simulink model "Modell_PADDELEC_RB_V3"  (R2019b)
settings: Solver=FixedStepAuto  StartTime=0.0  StopTime=269.98659999999654  FixedStep=0.1  RelTol=1e-3
model workspace (MAT data in the model file):
  SDO_OutputTimes = [0 0.00219999999536 0.0177999999942 0.0334999999977 0.0399999999936 0.0490999999965 0.0497999999934 0.0646999999954 0.0799999999945 0.0802999999942 0.0959000000003 0.111599999997 ... (25110 elements, 25110x1)]
values from neighbouring files (symbols this model uses):
  BAT = clsBattery    [start.m]
  BLDC = clsBLDC    [start.m]
  BoatHull = clsBoatHull    [start.m]
  MotorECU = clsMotorECU    [start.m]
libraries: fl_lib x51, nesl_utility x28, ee_lib x3, simulink x2, eeGeneralControl x1
(part 2 of 2)

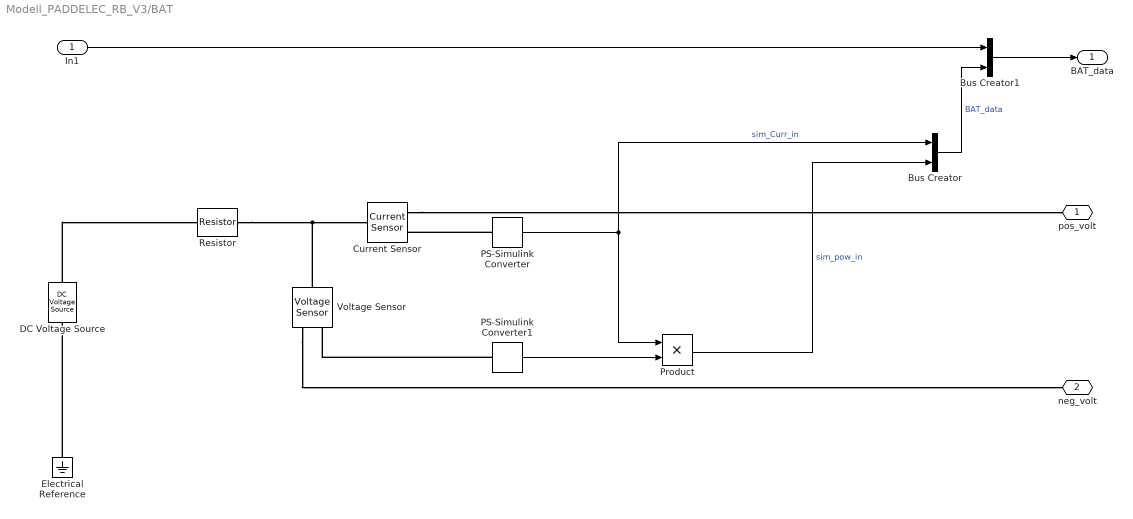
== system Modell_PADDELEC_RB_V3/BAT ==
  In1 : Inport
  Bus Creator : BusCreator  Inputs=2
  Bus Creator1 : BusCreator  Inputs=2
  Current Sensor : fl_lib/Electrical/Electrical Sensors/Current Sensor
  DC Voltage Source : fl_lib/Electrical/Electrical Sources/DC Voltage Source  v0=BAT.Voltage V
  Electrical Reference : fl_lib/Electrical/Electrical Elements/Electrical Reference
  PS-Simulink Converter : nesl_utility/PS-Simulink Converter  PhysicalDomain=network_engine_domain  SubClassName=ps_output  LeftPortType=input  RightPortType=output  PseudoPeriodic=off  Frequencies=[]  Unit=1  AffineConversion=off
  PS-Simulink Converter1 : nesl_utility/PS-Simulink Converter  PhysicalDomain=network_engine_domain  SubClassName=ps_output  LeftPortType=input  RightPortType=output  PseudoPeriodic=off  Frequencies=[]  Unit=1  AffineConversion=off
  Product : Product
  Resistor : fl_lib/Electrical/Electrical Elements/Resistor  R=BAT.InternalResistance Ohm  i_specify=off  i_priority=High  i=0 A  i_nominal_specify=off  i_nominal_unit=A  i_nominal_value=1  v_specify=off  v_priority=High  v=0 V  v_nominal_specify=off  v_nominal_unit=V  v_nominal_value=1
  Voltage Sensor : fl_lib/Electrical/Electrical Sensors/Voltage Sensor
  pos_volt : PMIOPort  Side=Right
  neg_volt : PMIOPort  Port=2  Side=Right
  BAT_data : Outport
  wires:
  PS-Simulink Converter/1 -> Product/1, Bus Creator/1  "sim_Curr_in"
  Product/1 -> Bus Creator/2  "sim_pow_in"
  PS-Simulink Converter1/1 -> Product/2
  Bus Creator1/1 -> BAT_data/1
  Bus Creator/1 -> Bus Creator1/2  "BAT_data"
  In1/1 -> Bus Creator1/1
  connections:
  Electrical Reference/LConn1 -- DC Voltage Source/RConn1
  Voltage Sensor/LConn1 -- Current Sensor/LConn1 -- Resistor/RConn1
  PS-Simulink Converter1/LConn1 -- Voltage Sensor/RConn1
  PS-Simulink Converter/LConn1 -- Current Sensor/RConn1
  DC Voltage Source/LConn1 -- Resistor/LConn1
  Voltage Sensor/RConn2 -- neg_volt/RConn1
  Current Sensor/RConn2 -- pos_volt/RConn1

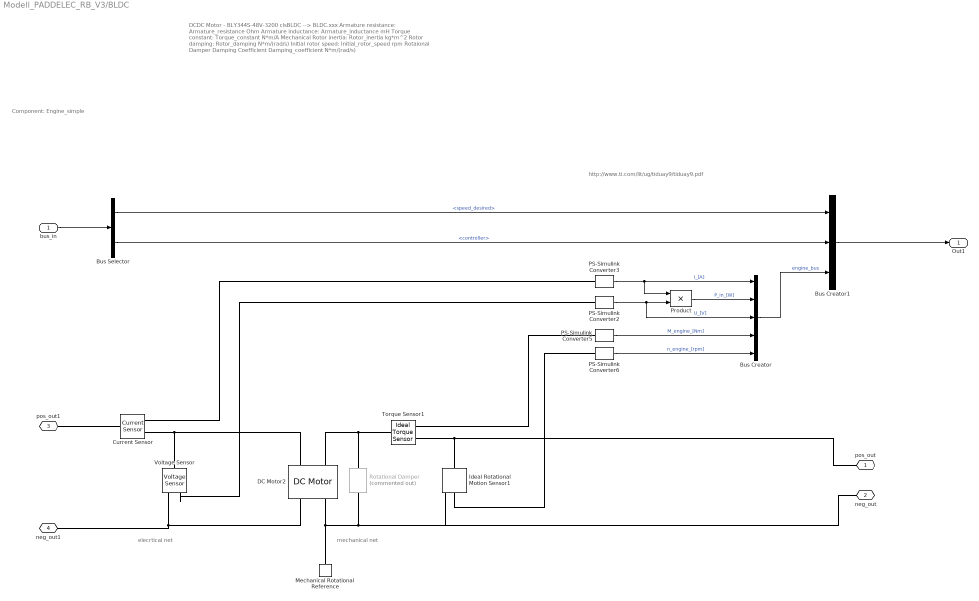
== system Modell_PADDELEC_RB_V3/BLDC ==
  note: http://www.ti.com/lit/ug/tiduay9/tiduay9.pdf
  note: mechanical net
  note: DCDC Motor - BLY344S-48V-3200
      |
      | clsBLDC --> BLDC.xxx
      |
      | Armature resistance:
      | Armature_resistance
      | Ohm
      |
      | Armature inductance:
      | Armature_inductance
      | mH
      |
      | Torque constant:
      | Torque_constant
      | N*m/A
      |
      | Mechanical
      |
      | Rotor inertia:
      | Rotor_inertia
      | kg*m^2
      |
      | Rotor damping:
      | Rotor_damping
      | N*m/(rad/s)
      |
      | Initial rotor speed:
      | Initial_rotor_speed
      | rpm
      |
      | Rotaional Damper
      |
      | Damping Coefficient
      | Damping_coefficient
      | N*m/(rad/s)
  note: elecrtical net
  note: Component:
      | Engine_simple
  bus_in : Inport
  Bus Creator : BusCreator  Inputs=5
  Bus Creator1 : BusCreator  Inputs=3
  Bus Selector : BusSelector  OutputSignals=speed_desired,controller
  Current Sensor : fl_lib/Electrical/Electrical Sensors/Current Sensor
  DC Motor2 : ee_lib/Electromechanical/Brushed Motors/DC Motor  parameterization=1  Ra=BLDC.Armature_resistance Ohm  La=BLDC.Armature_inductance mH  emf_or_torque=2  Kv=0.00907 V/rpm  Ki=BLDC.Torque_constant N*m/A  T_stall=3e-3*4000/(2*pi*6.25) N*m  w_max=3200 rpm  w_rated=3200 rpm  P_rated=660 W  V_rated=48 V  J="BLDC.Rotor_inertia  kg*m^2"  lam_param=1  lam=BLDC.Rotor_damping N*m/(rad/s)  i_noload=0 A  V_i_noload=1.5 V  speed0=BLDC.Initial_rotor_speed rpm  alpha=3.93e-3 1/K  Tmeas=25 degC  thermal_mass=100 J/K  initial_temperature=25 degC
      settings: SourceProductName=Simscape Electrical
  Ideal Rotational Motion Sensor1 : fl_lib/Mechanical/Mechanical Sensors/Ideal Rotational Motion Sensor  offset=0 rad
  Mechanical Rotational Reference : fl_lib/Mechanical/Rotational Elements/Mechanical Rotational Reference
  PS-Simulink Converter2 : nesl_utility/PS-Simulink Converter  PhysicalDomain=network_engine_domain  SubClassName=ps_output  LeftPortType=input  RightPortType=output  PseudoPeriodic=off  Frequencies=[]  Unit=V  AffineConversion=off
  PS-Simulink Converter3 : nesl_utility/PS-Simulink Converter  PhysicalDomain=network_engine_domain  SubClassName=ps_output  LeftPortType=input  RightPortType=output  PseudoPeriodic=off  Frequencies=[]  Unit=A  AffineConversion=off
  PS-Simulink Converter5 : nesl_utility/PS-Simulink Converter  PhysicalDomain=network_engine_domain  SubClassName=ps_output  LeftPortType=input  RightPortType=output  PseudoPeriodic=off  Frequencies=[]  Unit=N*m  AffineConversion=on
  PS-Simulink Converter6 : nesl_utility/PS-Simulink Converter  PhysicalDomain=network_engine_domain  SubClassName=ps_output  LeftPortType=input  RightPortType=output  PseudoPeriodic=off  Frequencies=[]  Unit=rpm  AffineConversion=on
  Product : Product
  Rotational Damper : fl_lib/Mechanical/Rotational Elements/Rotational Damper  Commented=on  D=2.5000e-04 N*m/(rad/s)  w_specify=off  w_priority=High  w=0 rad/s  w_nominal_specify=off  w_nominal_unit=rad/s  w_nominal_value=1  t_specify=off  t_priority=High  t=0 N*m  t_nominal_specify=off  t_nominal_unit=N*m  t_nominal_value=1
  Torque Sensor1 : fl_lib/Mechanical/Mechanical Sensors/Ideal Torque Sensor
  Voltage Sensor : fl_lib/Electrical/Electrical Sensors/Voltage Sensor
  pos_out : PMIOPort  Side=Right
  neg_out : PMIOPort  Port=2  Side=Right
  pos_out1 : PMIOPort  Port=3  Side=Left
  neg_out1 : PMIOPort  Port=4  Side=Left
  Out1 : Outport
  wires:
  Bus Creator1/1 -> Out1/1
  Bus Selector/2 -> Bus Creator1/2  "<controller>"
  Product/1 -> Bus Creator/2  "P_in_[W]"
  PS-Simulink Converter3/1 -> Bus Creator/1, Product/1  "I_[A]"
  bus_in/1 -> Bus Selector/1
  PS-Simulink Converter2/1 -> Bus Creator/3, Product/2  "U_[V]"
  Bus Creator/1 -> Bus Creator1/3  "engine_bus"
  PS-Simulink Converter5/1 -> Bus Creator/4  "M_engine_[Nm]"
  PS-Simulink Converter6/1 -> Bus Creator/5  "n_engine_[rpm]"
  Bus Selector/1 -> Bus Creator1/1  "<speed_desired>"
  connections:
  DC Motor2/RConn1 -- Voltage Sensor/RConn2 -- neg_out1/RConn1
  Torque Sensor1/RConn1 -- Ideal Rotational Motion Sensor1/LConn1 -- pos_out/RConn1
  DC Motor2/RConn2 -- Rotational Damper/RConn1 -- neg_out/RConn1 -- Ideal Rotational Motion Sensor1/RConn1 -- Mechanical Rotational Reference/LConn1
  DC Motor2/LConn2 -- Torque Sensor1/LConn1 -- Rotational Damper/LConn1
  DC Motor2/LConn1 -- Current Sensor/RConn2 -- Voltage Sensor/LConn1
  Ideal Rotational Motion Sensor1/RConn2 -- PS-Simulink Converter6/LConn1
  Torque Sensor1/RConn2 -- PS-Simulink Converter5/LConn1
  pos_out1/RConn1 -- Current Sensor/LConn1
  Voltage Sensor/RConn1 -- PS-Simulink Converter2/LConn1
  Current Sensor/RConn1 -- PS-Simulink Converter3/LConn1

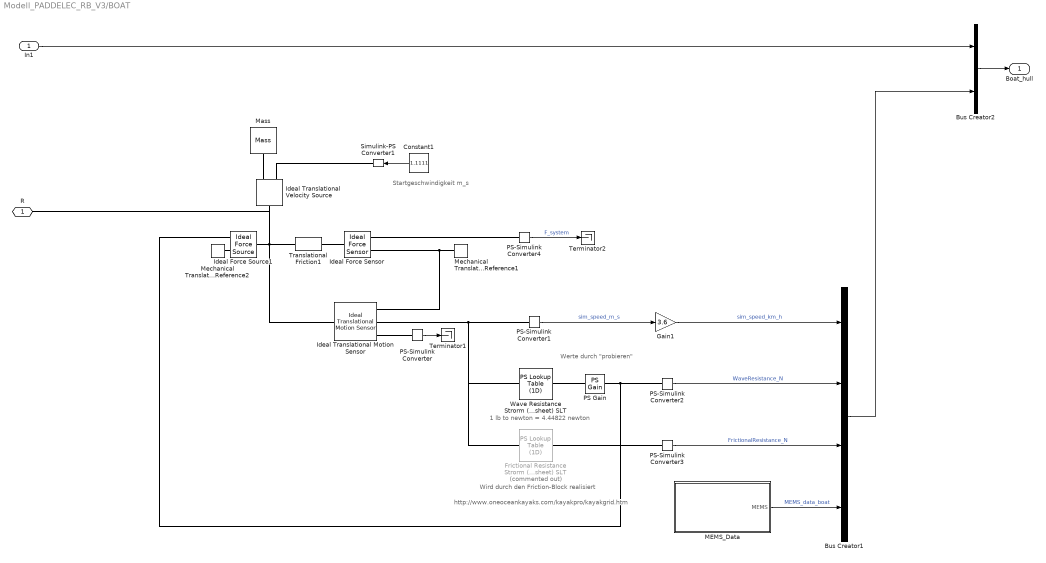
== system Modell_PADDELEC_RB_V3/BOAT ==
  note: Startgeschwindigkeit m_s
  note: Wird durch den Friction-Block realisiert
  note: 1 lb to newton = 4.44822 newton
  note: http://www.oneoceankayaks.com/kayakpro/kayakgrid.htm
  note: Werte durch "probieren"
  In1 : Inport
  Bus Creator1 : BusCreator  Inputs=4
  Bus Creator2 : BusCreator  Inputs=2
  Constant1 : Constant  Value=1.1111
  Frictional Resistance Strorm (datasheet) SLT : fl_lib/Physical Signals/Lookup Tables/PS Lookup Table (1D)  Commented=on  x=SpeedVec_m_s m/s  f=FricResistance_N  interp_method=simscape.enum.interpolation.smooth  extrap_method=simscape.enum.extrapolation.linear
      settings: SourceProductName=Simscape  SourceProductBaseCode=SS
  Gain1 : Gain  Gain=3.6
  Ideal Force Sensor : fl_lib/Mechanical/Mechanical Sensors/Ideal Force Sensor
  Ideal Force Source1 : fl_lib/Mechanical/Mechanical Sources/Ideal Force Source
  Ideal Translational Motion Sensor : fl_lib/Mechanical/Mechanical Sensors/Ideal Translational Motion Sensor  offset=0 m
  Ideal Translational Velocity Source : fl_lib/Mechanical/Mechanical Sources/Ideal Translational Velocity Source
  MEMS_Data : Subsystem
      mask Display: image('D:\00_Sandbox\Matlab\Modell_20200324\03_symbols\Lagesensoren.png'); % Use "Edit Image" on toolstrip to change.
  Mass : fl_lib/Mechanical/Translational Elements/Mass  mass=BoatHull.Mass + 195.5 kg  v_specify=off  v_priority=High  v=0 m/s  v_nominal_specify=off  v_nominal_unit=m/s  v_nominal_value=1  f_specify=off  f_priority=None  f=0 N  f_nominal_specify=off  f_nominal_unit=N  f_nominal_value=1
  Mechanical Translational Reference1 : fl_lib/Mechanical/Translational Elements/Mechanical Translational Reference
  Mechanical Translational Reference2 : fl_lib/Mechanical/Translational Elements/Mechanical Translational Reference
  PS Gain : fl_lib/Physical Signals/Functions/PS Gain  gain=-32
  PS-Simulink Converter : nesl_utility/PS-Simulink Converter  PhysicalDomain=network_engine_domain  SubClassName=ps_output  LeftPortType=input  RightPortType=output  PseudoPeriodic=off  Frequencies=[]  Unit=inherit  AffineConversion=off
  PS-Simulink Converter1 : nesl_utility/PS-Simulink Converter  PhysicalDomain=network_engine_domain  SubClassName=ps_output  LeftPortType=input  RightPortType=output  PseudoPeriodic=off  Frequencies=[]  Unit=inherit  AffineConversion=off
  PS-Simulink Converter2 : nesl_utility/PS-Simulink Converter  PhysicalDomain=network_engine_domain  SubClassName=ps_output  LeftPortType=input  RightPortType=output  PseudoPeriodic=off  Frequencies=[]  Unit=inherit  AffineConversion=on
  PS-Simulink Converter3 : nesl_utility/PS-Simulink Converter  PhysicalDomain=network_engine_domain  SubClassName=ps_output  LeftPortType=input  RightPortType=output  PseudoPeriodic=off  Frequencies=[]  Unit=inherit  AffineConversion=on
  PS-Simulink Converter4 : nesl_utility/PS-Simulink Converter  PhysicalDomain=network_engine_domain  SubClassName=ps_output  LeftPortType=input  RightPortType=output  PseudoPeriodic=off  Frequencies=[]  Unit=inherit  AffineConversion=off
  Simulink-PS Converter1 : nesl_utility/Simulink-PS Converter  PhysicalDomain=network_engine_domain  SubClassName=ps_input  LeftPortType=input  RightPortType=output  PseudoPeriodic=off  Frequencies=[]  NoiseDistribution=none  NoiseParameters=[]  Unit=1  AffineConversion=off  FilteringAndDerivatives=provide  SimscapeFilterOrder=1  InputFilterTimeConstant=0.001  UdotUserProvided=0
  Terminator1 : Terminator
  Terminator2 : Terminator
  Translational Friction1 : fl_lib/Mechanical/Translational Elements/Translational Friction  brkwy_frc=BoatHull.BreakawayFrictionForce N  brkwy_vel=BoatHull.BreakawayFrictionVelocity m/s  Col_frc=BoatHull.ColumbFrictionForce N  visc_coef=BoatHull.ViscousFriction N/(m/s)  v_specify=off  v_priority=None  v=0 m/s  v_nominal_specify=off  v_nominal_unit=m/s  v_nominal_value=1  f_specify=off  f_priority=None  f=0 N  f_nominal_specify=off  f_nominal_unit=N  f_nominal_value=1
      settings: SourceProductName=Simscape  SourceProductBaseCode=SS  InternalSimscapePortConfiguration="{\"Bottom\":[],\"Left\":[{\"id\":\"R\",\"label\":\"R\",\"type\":\"foundation.mechanical.translational.translational\"}],\"Right\":[{\"id\":\"C\",\"label\":\"C\",\"type\":\"foundation.mechanical.translational.translational\"}],\"Top\":[]}"
  Wave Resistance Strorm (datasheet) SLT : fl_lib/Physical Signals/Lookup Tables/PS Lookup Table (1D)  x=BoatHull.SpeedVec_m_s m/s  f=BoatHull.WaveResistance_N  interp_method=simscape.enum.interpolation.smooth  extrap_method=simscape.enum.extrapolation.linear
      settings: SourceProductName=Simscape  SourceProductBaseCode=SS
  R : PMIOPort  Side=Left
  Boat_hull : Outport  VectorParamsAs1DForOutWhenUnconnected=off
  wires:
  PS-Simulink Converter/1 -> Terminator1/1
  PS-Simulink Converter2/1 -> Bus Creator1/2  "WaveResistance_N"
  Gain1/1 -> Bus Creator1/1  "sim_speed_km_h"
  PS-Simulink Converter1/1 -> Gain1/1  "sim_speed_m_s"
  PS-Simulink Converter3/1 -> Bus Creator1/3  "FrictionalResistance_N"
  PS-Simulink Converter4/1 -> Terminator2/1  "F_system"
  Constant1/1 -> Simulink-PS Converter1/1
  MEMS_Data/1(MEMS) -> Bus Creator1/4  "MEMS_data_boat"
  In1/1 -> Bus Creator2/1
  Bus Creator1/1 -> Bus Creator2/2
  Bus Creator2/1 -> Boat_hull/1
  connections:
  Ideal Translational Motion Sensor/LConn1 -- R/RConn1 -- Ideal Translational Velocity Source/LConn1 -- Ideal Force Source1/LConn1 -- Translational Friction1/LConn1
  Ideal Translational Motion Sensor/RConn1 -- Mechanical Translational Reference1/LConn1 -- Ideal Force Sensor/RConn1
  PS-Simulink Converter/LConn1 -- Ideal Translational Motion Sensor/RConn3
  Ideal Translational Motion Sensor/RConn2 -- Frictional Resistance Strorm (datasheet) SLT/LConn1 -- Wave Resistance Strorm (datasheet) SLT/LConn1 -- PS-Simulink Converter1/LConn1
  PS-Simulink Converter3/LConn1 -- Frictional Resistance Strorm (datasheet) SLT/RConn1
  PS-Simulink Converter2/LConn1 -- Ideal Force Source1/RConn1 -- PS Gain/RConn1
  PS Gain/LConn1 -- Wave Resistance Strorm (datasheet) SLT/RConn1
  PS-Simulink Converter4/LConn1 -- Ideal Force Sensor/RConn2
  Ideal Force Sensor/LConn1 -- Translational Friction1/RConn1
  Simulink-PS Converter1/RConn1 -- Ideal Translational Velocity Source/RConn1
  Ideal Translational Velocity Source/RConn2 -- Mass/LConn1
  Mechanical Translational Reference2/LConn1 -- Ideal Force Source1/RConn2

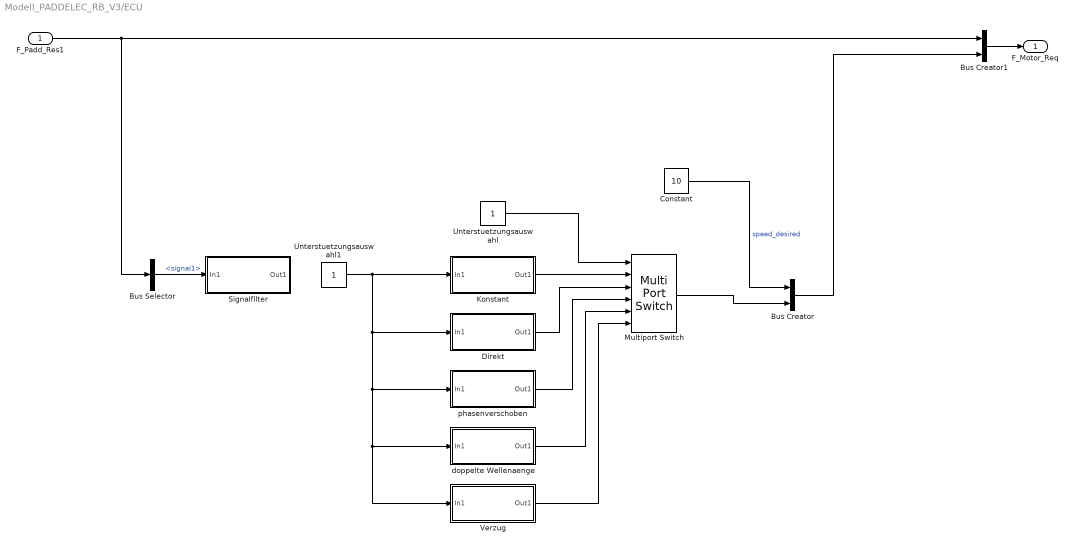
== system Modell_PADDELEC_RB_V3/ECU ==
  F_Padd_Res1 : Inport
  Bus Creator : BusCreator  Inputs=2
  Bus Creator1 : BusCreator  Inputs=2
  Bus Selector : BusSelector  OutputSignals=signal1
  Constant : Constant  Value=10
  Direkt : Subsystem
  Konstant : Subsystem
  Multiport Switch : MultiPortSwitch  Inputs=5
  Signalfilter : Subsystem
  Unterstuetzungsauswahl : Constant
  Unterstuetzungsauswahl1 : Constant
  Verzug : Subsystem
  doppelte Wellenaenge : Subsystem
  phasenverschoben : Subsystem
  F_Motor_Req : Outport  VectorParamsAs1DForOutWhenUnconnected=off
  wires:
  Konstant/1(Out1) -> Multiport Switch/2
  Unterstuetzungsauswahl1/1 -> Verzug/1(In1), doppelte Wellenaenge/1(In1), phasenverschoben/1(In1), Direkt/1(In1), Konstant/1(In1)
  Direkt/1(Out1) -> Multiport Switch/3
  Unterstuetzungsauswahl/1 -> Multiport Switch/1
  phasenverschoben/1(Out1) -> Multiport Switch/4
  doppelte Wellenaenge/1(Out1) -> Multiport Switch/5
  Verzug/1(Out1) -> Multiport Switch/6
  Constant/1 -> Bus Creator/1  "speed_desired"
  Multiport Switch/1 -> Bus Creator/2
  F_Padd_Res1/1 -> Bus Creator1/1, Bus Selector/1
  Bus Creator/1 -> Bus Creator1/2
  Bus Creator1/1 -> F_Motor_Req/1
  Bus Selector/1 -> Signalfilter/1(In1)  "<signal1>"

== system Modell_PADDELEC_RB_V3/JET  ==
  n_Motor : Inport
  Mechanical Rotational Reference : fl_lib/Mechanical/Rotational Elements/Mechanical Rotational Reference
  Slider-Crank : fl_lib/Mechanical/Mechanisms/Slider-Crank  crank=.1 m  rod=.2 m  inertia=0.01 kg*m^2  k=1e6 N/m  b=1e3 N/(m/s)  theta_specify=off  theta_priority=High  theta=1.570796326794897 rad  theta_nominal_specify=off  theta_nominal_unit=rad  theta_nominal_value=1  w_specify=off  w_priority=High  w=0 rad/s  w_nominal_specify=off  w_nominal_unit=rad/s  w_nominal_value=1
      settings: SourceProductName=Simscape  SourceProductBaseCode=SS  InternalSimscapePortConfiguration="{\"Bottom\":[],\"Left\":[{\"id\":\"C\",\"label\":\"C\",\"type\":\"foundation.mechanical.rotational.rotational\"}],\"Right\":[{\"id\":\"S\",\"label\":\"S\",\"type\":\"foundation.mechanical.translational.translational\"}],\"Top\":[]}"
  pos_in : PMIOPort  Side=Left
  R : PMIOPort  Port=2  Side=Right
  neg_in : PMIOPort  Port=3  Side=Left
  F_Jet : Outport
  wires:
  n_Motor/1 -> F_Jet/1
  connections:
  pos_in/RConn1 -- Slider-Crank/LConn1
  Slider-Crank/RConn1 -- R/RConn1
  neg_in/RConn1 -- Mechanical Rotational Reference/LConn1

== system Modell_PADDELEC_RB_V3/Messungen ==
  Bus Creator : BusCreator  Inputs=2
  From Workspace1 : FromWorkspace  VariableName=tsc_paddel4.scaledAccelX  SampleTime=0
  From Workspace2 : FromWorkspace  VariableName=tsc_paddel4.speed  SampleTime=0
  Gain : Gain  Gain=-1
  Gain1 : Gain  Gain=3.6
  measurement_data : Outport
  wires:
  From Workspace1/1 -> Gain/1
  Gain/1 -> Bus Creator/1  "a_Boat"
  From Workspace2/1 -> Gain1/1  "v_Boat"
  Bus Creator/1 -> measurement_data/1
  Gain1/1 -> Bus Creator/2  "v_Boat_km_h"

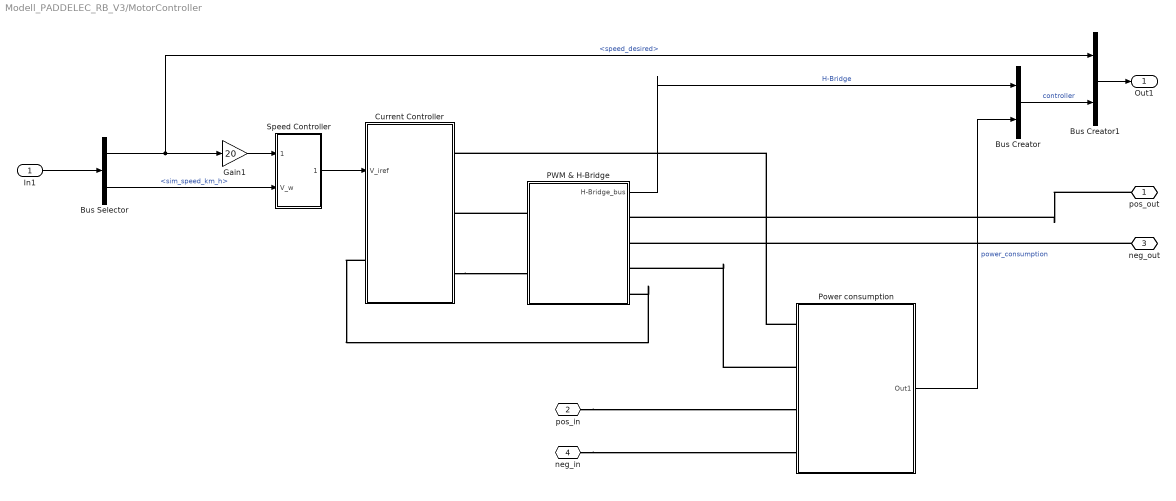
== system Modell_PADDELEC_RB_V3/MotorController ==
  In1 : Inport
  Bus Creator : BusCreator  Inputs=2
  Bus Creator1 : BusCreator  Inputs=2
  Bus Selector : BusSelector  OutputSignals=signal1.signal2.speed_desired,signal1.signal1.signal1.signal2.sim_speed_km_h
  Current Controller : Subsystem
  Gain1 : Gain  Gain=20
  PWM & H-Bridge : Subsystem
  Power consumption : Subsystem
  Speed Controller : Subsystem  VariantControl=VSS_SpeedController_simple
  pos_out : PMIOPort  Side=Right
  pos_in : PMIOPort  Port=2  Side=Left
  neg_out : PMIOPort  Port=3  Side=Right
  neg_in : PMIOPort  Port=4  Side=Left
  Out1 : Outport
  wires:
  In1/1 -> Bus Selector/1
  Power consumption/1(Out1) -> Bus Creator/2  "power_consumption"
  Gain1/1 -> Speed Controller/1(V_wref)
  Bus Creator1/1 -> Out1/1
  Bus Selector/2 -> Speed Controller/2(V_w)  "<sim_speed_km_h>"
  Speed Controller/1(V_iref) -> Current Controller/1(V_iref)
  PWM & H-Bridge/1(H-Bridge_bus) -> Bus Creator/1  "H-Bridge"
  Bus Creator/1 -> Bus Creator1/2  "controller"
  Bus Selector/1 -> Gain1/1, Bus Creator1/1  "<speed_desired>"
  connections:
  neg_out/RConn1 -- PWM & H-Bridge/RConn2
  PWM & H-Bridge/LConn1 -- Current Controller/RConn2
  Current Controller/RConn3 -- PWM & H-Bridge/LConn2
  pos_out/RConn1 -- PWM & H-Bridge/RConn1
  Power consumption/LConn2 -- PWM & H-Bridge/RConn3
  Power consumption/LConn1 -- Current Controller/RConn1
  Current Controller/LConn1 -- PWM & H-Bridge/RConn4
  pos_in/RConn1 -- Power consumption/LConn3
  neg_in/RConn1 -- Power consumption/LConn4

== system Modell_PADDELEC_RB_V3/Subsystem1 ==
  a_Boat_sim : Inport
  In4 : Inport  Port=2
  Bus Selector : BusSelector  OutputSignals=signal2.sim_speed_km_h,signal2.WaveResistance_N
  Bus Selector1 : BusSelector  OutputSignals=a_Boat,v_Boat_km_h
  v_Boat : Scope  NumInputPorts=2
  v_Boat1 : Scope  NumInputPorts=2
  wires:
  a_Boat_sim/1 -> Bus Selector/1
  In4/1 -> Bus Selector1/1
  Bus Selector/1 -> v_Boat/1  "<sim_speed_km_h>"
  Bus Selector/2 -> v_Boat/2  "<WaveResistance_N>"
  Bus Selector1/1 -> v_Boat1/1  "<a_Boat>"
  Bus Selector1/2 -> v_Boat1/2  "<v_Boat_km_h>"

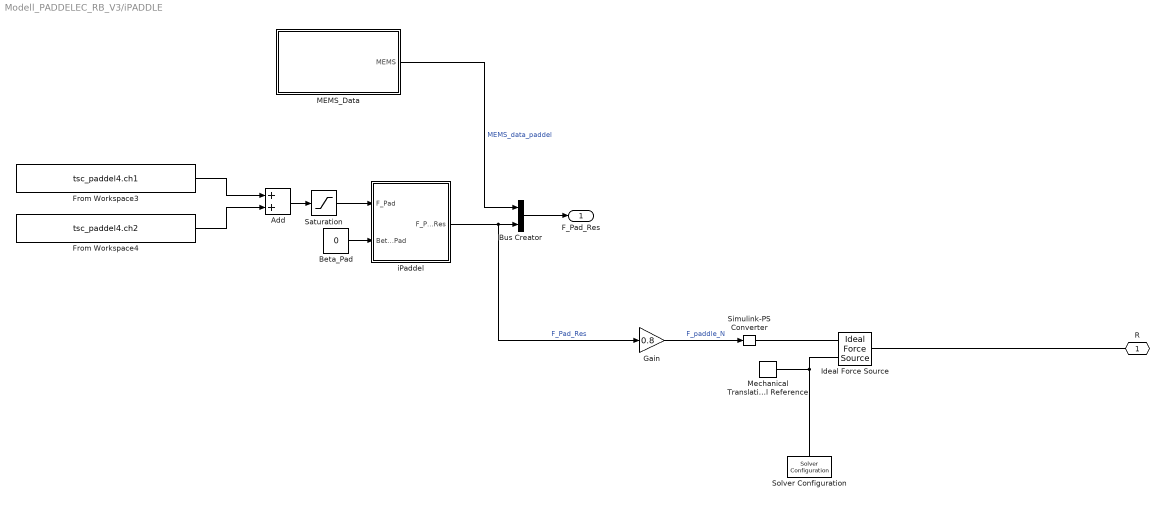
== system Modell_PADDELEC_RB_V3/iPADDLE ==
  Add : Sum
  Beta_Pad : Constant  Value=0
  Bus Creator : BusCreator  Inputs=2
  From Workspace3 : FromWorkspace  VariableName=tsc_paddel4.ch1  SampleTime=0
  From Workspace4 : FromWorkspace  VariableName=tsc_paddel4.ch2  SampleTime=0
  Gain : Gain  Gain=0.8
  Ideal Force Source : fl_lib/Mechanical/Mechanical Sources/Ideal Force Source
  MEMS_Data : Subsystem
      mask Display: image('D:\00_Sandbox\Matlab\Modell_20200324\03_symbols\Lagesensoren.png'); % Use "Edit Image" on toolstrip to change.
  Mechanical Translational Reference : fl_lib/Mechanical/Translational Elements/Mechanical Translational Reference
  Saturation : Saturate  UpperLimit=inf  LowerLimit=0
  Simulink-PS Converter : nesl_utility/Simulink-PS Converter  PhysicalDomain=network_engine_domain  SubClassName=ps_input  LeftPortType=input  RightPortType=output  PseudoPeriodic=off  Frequencies=[]  NoiseDistribution=none  NoiseParameters=[]  Unit=1  AffineConversion=off  FilteringAndDerivatives=provide  SimscapeFilterOrder=1  InputFilterTimeConstant=0.001  UdotUserProvided=0
  Solver Configuration : nesl_utility/Solver Configuration  PhysicalDomain=network_engine_domain  SubClassName=solver  LeftPortType=input  RightPortType=generic  Tones=[]  Harmonics=[]  SimulateNoise=off  Profile=off  UseLocalSampling=off  EnableSwitchedLinearOptims=on  FrequencyDomain=off  UseCCode=off  RelTol=0.001  AbsTol=1e-06  MinStep=1e-09  ToWorkspace=off  RevertToSquareIcSolve=off  NumHomotopyIterations=100  PhasorMode=off  PhasorModeNumHarmonics=1  DoDC=off  ResidualTolerance=1e-09  UseLocalSolver=off  LocalSolverChoice=NE_BACKWARD_EULER_ADVANCER  LocalSolverSampleTime=0.001  DoFixedCost=off  MaxNonlinIter=3  MaxModeIter=2  LinearAlgebra=auto  EquationFormulation=NE_TIME_EF  DelaysMemoryBudget=1024  AutomaticFiltering=on  FilteringTimeConstant=0.001  PartitionStorageMethod=AS_NEEDED  PartitionMemoryBudget=1024  PartitionMethod=ROBUST
  iPaddel : Subsystem
  R : PMIOPort  Side=Right
  F_Pad_Res : Outport
  wires:
  Beta_Pad/1 -> iPaddel/2(Beta_Pad)
  Add/1 -> Saturation/1
  From Workspace3/1 -> Add/1
  From Workspace4/1 -> Add/2
  Bus Creator/1 -> F_Pad_Res/1
  iPaddel/1(F_Pad_Res) -> Gain/1, Bus Creator/2  "F_Pad_Res"
  Saturation/1 -> iPaddel/1(F_Pad)
  Gain/1 -> Simulink-PS Converter/1  "F_paddle_N"
  MEMS_Data/1(MEMS) -> Bus Creator/1  "MEMS_data_paddel"
  connections:
  Mechanical Translational Reference/LConn1 -- Solver Configuration/RConn1 -- Ideal Force Source/RConn2
  Simulink-PS Converter/RConn1 -- Ideal Force Source/RConn1
  Ideal Force Source/LConn1 -- R/RConn1

== system Modell_PADDELEC_RB_V3/BOAT/MEMS_Data ==
  Beta_Pad : Constant  Value=0
  Bus Creator : BusCreator  Inputs=1
  MEMS : Outport
  wires:
  Beta_Pad/1 -> Bus Creator/1
  Bus Creator/1 -> MEMS/1

== system Modell_PADDELEC_RB_V3/ECU/Direkt ==
  In1 : Inport
  Out1 : Outport
  wires:
  In1/1 -> Out1/1

== system Modell_PADDELEC_RB_V3/ECU/Konstant ==
  In1 : Inport
  Moving Average : eeGeneralControl/Moving Average  VariantControl=Variant1  LabelModeActiveChoice=Continuous  f=0.08  x0=0  Ts=0
      settings: SourceProductName=Simscape Electrical  SourceProductBaseCode=PS
  Out1 : Outport
  wires:
  In1/1 -> Moving Average/1
  Moving Average/1 -> Out1/1

== system Modell_PADDELEC_RB_V3/ECU/Signalfilter ==
  In1 : Inport
  Out1 : Outport
  wires:
  In1/1 -> Out1/1

== system Modell_PADDELEC_RB_V3/ECU/Verzug ==
  In1 : Inport
  Out1 : Outport
  wires:
  In1/1 -> Out1/1

== system Modell_PADDELEC_RB_V3/ECU/doppelte Wellenaenge ==
  In1 : Inport
  Out1 : Outport
  wires:
  In1/1 -> Out1/1

== system Modell_PADDELEC_RB_V3/ECU/phasenverschoben ==
  In1 : Inport
  Out1 : Outport
  wires:
  In1/1 -> Out1/1

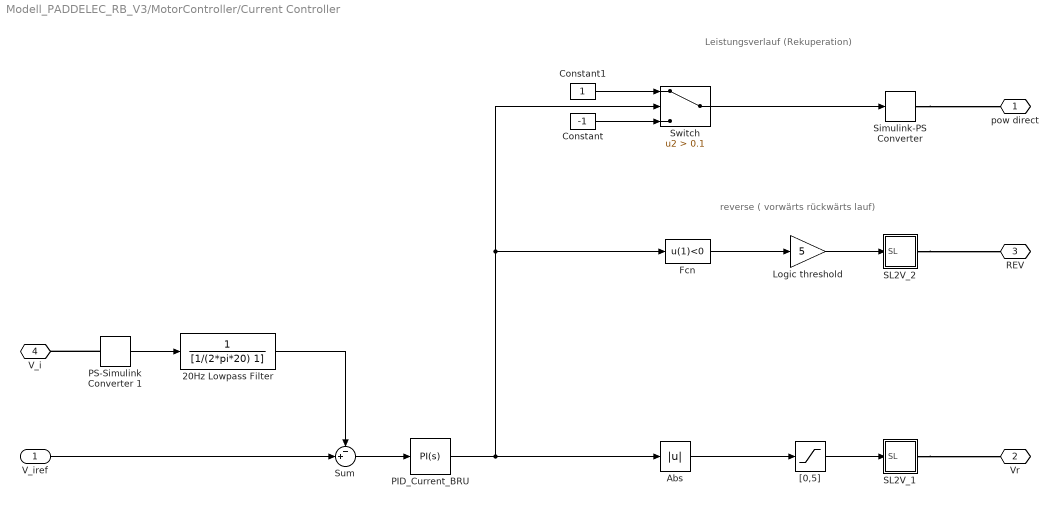
== system Modell_PADDELEC_RB_V3/MotorController/Current Controller ==
  note: reverse ( vorwärts rückwärts lauf)
  note: Leistungsverlauf (Rekuperation)
  V_iref : Inport
  20Hz Lowpass Filter : TransferFcn  Denominator=[1/(2*pi*20) 1]
  Abs : Abs
  Constant : Constant  Value=-1
  Constant1 : Constant
  Fcn : Fcn  Expr=u(1)<0
  Logic threshold : Gain  Gain=5
  PID_Current_BRU : simulink/Continuous/PID Controller  Controller=PI  Form=Parallel  TimeDomain=Continuous-time  SampleTime=-1  IntegratorMethod=Forward Euler  FilterMethod=Forward Euler  ControllerParametersSource=internal  P=MotorECU.Current_Prop  I=MotorECU.Current_Int  D=0  UseFilter=on  N=100  TunerSelectOption=Transfer Function Based (PID Tuner App)  InitialConditionSource=internal  InitialConditionForIntegrator=0  InitialConditionForFilter=0  DifferentiatorICPrevScaledInput=0  ExternalReset=none  TrackingMode=off  Kt=1  LimitOutput=off  UpperSaturationLimit=1.71  LowerSaturationLimit=-5  LinearizeAsGain=on  AntiWindupMode=back-calculation  Kb=1  POutMin=[]  POutMax=[]  IOutMin=[]  IOutMax=[]  DOutMin=[]  DOutMax=[]  NOutMin=[]  NOutMax=[]  SumOutMin=[]  SumOutMax=[]  SaturationOutMin=[]  SaturationOutMax=[]  PParamMin=[]  PParamMax=[]  IParamMin=[]  IParamMax=[]  DParamMin=[]  DParamMax=[]  NParamMin=[]  NParamMax=[]  KbParamMin=[]  KbParamMax=[]  KtParamMin=[]  KtParamMax=[]  KbOutMin=[]  KbOutMax=[]  KtOutMin=[]  KtOutMax=[]  IntegratorOutMin=[]  IntegratorOutMax=[]  FilterOutMin=[]  FilterOutMax=[]  SumI1OutMin=[]  SumI1OutMax=[]  SumI2OutMin=[]  SumI2OutMax=[]  SumI3OutMin=[]  SumI3OutMax=[]  SumI4OutMin=[]  SumI4OutMax=[]  SumDOutMin=[]  SumDOutMax=[]  DifferentiatorOutMin=[]  DifferentiatorOutMax=[]  FilterDiffOutCoefMin=[]  FilterDiffOutCoefMax=[]  ReciprocalOutMin=[]  ReciprocalOutMax=[]  SumDenOutMin=[]  SumDenOutMax=[]  SumNumOutMin=[]  SumNumOutMax=[]  DivideOutMin=[]  DivideOutMax=[]  IntegratorContinuousStateAttributes=''  IntegratorStateMustResolveToSignalObject=off  IntegratorRTWStateStorageClass=Auto  FilterContinuousStateAttributes=''  FilterStateMustResolveToSignalObject=off  FilterRTWStateStorageClass=Auto  ParallelPVariant=InternalParameters  IdealPVariant=Disabled  IVariant=InternalParameters  DVariant=Disabled  IntegratorVariant=Continuous  SatVariant=Disabled  AWVariant=Passthrough  PCopyVariant=Disabled  TRVariant=Disabled  FdbkBlocksVariant=Forward  IdealPFdbkVariant=Disabled  SatFdbkVariant=Disabled  DerivativeFilterVariant=Disabled  NVariant=Disabled  NCopyVariant=Disabled_SignalSpec  FilterICVariant=Disabled  IntegratorICVariant=InternalICs  ExternalResetVariant=Disabled  TRSumVariant=Passthrough  SumFdbkVariant=Disabled  SumVariant=Sum_PI
  PS-Simulink Converter 1 : nesl_utility/PS-Simulink Converter  PhysicalDomain=network_engine_domain  SubClassName=ps_output  LeftPortType=input  RightPortType=output  PseudoPeriodic=off  Frequencies=[]  Unit=A  AffineConversion=off
  SL2V_1 : Subsystem
  SL2V_2 : Subsystem
  Simulink-PS Converter : nesl_utility/Simulink-PS Converter  PhysicalDomain=network_engine_domain  SubClassName=ps_input  LeftPortType=input  RightPortType=output  PseudoPeriodic=off  Frequencies=[]  NoiseDistribution=none  NoiseParameters=[]  Unit=1  AffineConversion=off  FilteringAndDerivatives=zero  SimscapeFilterOrder=1  InputFilterTimeConstant=0.001  UdotUserProvided=1
  Sum : Sum  Inputs=-+|
  Switch : Switch  Criteria=u2 > Threshold  Threshold=0.1
  "[0,5]" : Saturate  UpperLimit=5  LowerLimit=0
  pow direct : PMIOPort  Side=Right
  Vr : PMIOPort  Port=2  Side=Right
  REV : PMIOPort  Port=3  Side=Right
  V_i : PMIOPort  Port=4  Side=Left
  wires:
  "[0,5]"/1 -> SL2V_1/1(SL)
  Fcn/1 -> Logic threshold/1
  Abs/1 -> "[0,5]"/1
  20Hz Lowpass Filter/1 -> Sum/1
  V_iref/1 -> Sum/2
  Logic threshold/1 -> SL2V_2/1(SL)
  PID_Current_BRU/1 -> Switch/2, Fcn/1, Abs/1
  Sum/1 -> PID_Current_BRU/1
  Constant/1 -> Switch/3
  Constant1/1 -> Switch/1
  Switch/1 -> Simulink-PS Converter/1
  PS-Simulink Converter 1/1 -> 20Hz Lowpass Filter/1
  connections:
  SL2V_2/RConn1 -- REV/RConn1
  SL2V_1/RConn1 -- Vr/RConn1
  Simulink-PS Converter/RConn1 -- pow direct/RConn1
  PS-Simulink Converter 1/LConn1 -- V_i/RConn1

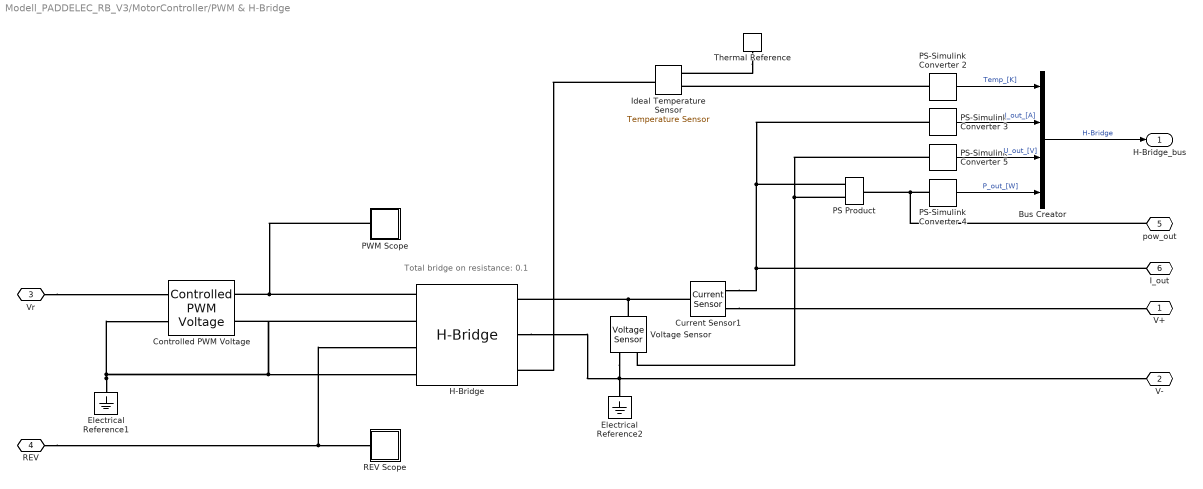
== system Modell_PADDELEC_RB_V3/MotorController/PWM & H-Bridge ==
  note: Total bridge on resistance: 0.1
  Bus Creator : BusCreator  Inputs=4
  Controlled PWM Voltage : ee_lib/Integrated Circuits/Controlled PWM Voltage  F=10000 Hz  TD=0 s  pulse_width_offset=0 s  pulse_min=0 s  Vmin=0 V  Vmax=5 V  Vm=5 V  pwm_or_av=2  event_type=1  sample_time=1e-6 s  u_min=0  u_max=1
      settings: SourceProductName=Simscape Electrical
  Current Sensor1 : fl_lib/Electrical/Electrical Sensors/Current Sensor
  Electrical Reference1 : fl_lib/Electrical/Electrical Elements/Electrical Reference
  Electrical Reference2 : fl_lib/Electrical/Electrical Elements/Electrical Reference
  H-Bridge : ee_lib/Semiconductors & Converters/Converters/H-Bridge  supply_ports=ee.enum.supply_ports.hidesupply  Venable=2.5 V  Vmax=5 V  Vreverse=2.5 V  Vbrake=2.5 V  Vm=500 V  pwm_or_av=2  regenerative_braking_mode=2  discontinuous=0  freewheeling_mode=1  Ron=10 Ohm  Don=0.1 Ohm  Goff=1e-6 S  Rload=10 Ohm  Lload=1e-5 H  F=10 kHz  thermal_mass=100 J/K  initial_temperature=298.15 K  Ron2=0.1 Ohm  Don2=0.05 Ohm  Tmeas=298.15 K  Tmeas2=398.15 K
      settings: SourceProductName=Simscape Electrical  LogSimulationData=on  InternalSimscapePortConfiguration="{\"Bottom\":[],\"Left\":[{\"id\":\"ENA\",\"label\":\"PWM\",\"type\":\"foundation.electrical.electrical\"},{\"id\":\"REF\",\"label\":\"REF\",\"type\":\"foundation.electrical.electrical\"},{\"id\":\"REV\",\"label\":\"REV\",\"type\":\"foundation.electrical.electrical\"},{\"id\":\"BRK\",\"label\":\"BRK\",\"type\":\"foundation.electrical.electrical\"}],\"Right\":[{\"id\":\"p2\",\"label\":\"+\",\"type\":\"foundation.electrical.electrical\"},{\"id\":\"n2\",\"label\":\"-\",\"type\":\"foundation.electrical.electrical\"},{\"id\":\"H\",\"label\":\"H\",\"type\":\"foundation.thermal.thermal\"}],\"Top\":[]}"
  Ideal Temperature Sensor : fl_lib/Thermal/Thermal Sensors/Temperature Sensor
  PS Product : fl_lib/Physical Signals/Functions/PS Product
      settings: SourceProductName=Simscape
  PS-Simulink Converter 2 : nesl_utility/PS-Simulink Converter  PhysicalDomain=network_engine_domain  SubClassName=ps_output  LeftPortType=input  RightPortType=output  PseudoPeriodic=off  Frequencies=[]  Unit=K  AffineConversion=off
  PS-Simulink Converter 3 : nesl_utility/PS-Simulink Converter  PhysicalDomain=network_engine_domain  SubClassName=ps_output  LeftPortType=input  RightPortType=output  PseudoPeriodic=off  Frequencies=[]  Unit=A  AffineConversion=off
  PS-Simulink Converter 4 : nesl_utility/PS-Simulink Converter  PhysicalDomain=network_engine_domain  SubClassName=ps_output  LeftPortType=input  RightPortType=output  PseudoPeriodic=off  Frequencies=[]  Unit=W  AffineConversion=off
  PS-Simulink Converter 5 : nesl_utility/PS-Simulink Converter  PhysicalDomain=network_engine_domain  SubClassName=ps_output  LeftPortType=input  RightPortType=output  PseudoPeriodic=off  Frequencies=[]  Unit=V  AffineConversion=off
  PWM Scope : Subsystem
  REV Scope : Subsystem
  Thermal Reference : fl_lib/Thermal/Thermal Elements/Thermal Reference
  Voltage Sensor : fl_lib/Electrical/Electrical Sensors/Voltage Sensor
  V+ : PMIOPort  Side=Right
  V- : PMIOPort  Port=2  Side=Right
  Vr : PMIOPort  Port=3  Side=Left
  REV : PMIOPort  Port=4  Side=Left
  pow_out : PMIOPort  Port=5  Side=Right
  I_out : PMIOPort  Port=6  Side=Right
  H-Bridge_bus : Outport
  wires:
  PS-Simulink Converter 2/1 -> Bus Creator/1  "Temp_[K]"
  Bus Creator/1 -> H-Bridge_bus/1  "H-Bridge"
  PS-Simulink Converter 3/1 -> Bus Creator/2  "I_out_[A]"
  PS-Simulink Converter 5/1 -> Bus Creator/3  "U_out_[V]"
  PS-Simulink Converter 4/1 -> Bus Creator/4  "P_out_[W]"
  connections:
  REV/RConn1 -- H-Bridge/LConn3 -- REV Scope/LConn1
  Vr/RConn1 -- Controlled PWM Voltage/LConn1
  Electrical Reference1/LConn1 -- Controlled PWM Voltage/LConn2 -- H-Bridge/LConn4 -- H-Bridge/LConn2 -- Controlled PWM Voltage/RConn2
  H-Bridge/LConn1 -- PWM Scope/LConn1 -- Controlled PWM Voltage/RConn1
  Voltage Sensor/RConn2 -- V-/RConn1 -- Electrical Reference2/LConn1 -- H-Bridge/RConn2
  Current Sensor1/LConn1 -- Voltage Sensor/LConn1 -- H-Bridge/RConn1
  PS-Simulink Converter 2/LConn1 -- Ideal Temperature Sensor/RConn2
  Ideal Temperature Sensor/LConn1 -- H-Bridge/RConn3
  Thermal Reference/LConn1 -- Ideal Temperature Sensor/RConn1
  PS Product/LConn2 -- PS-Simulink Converter 5/LConn1 -- Voltage Sensor/RConn1
  Current Sensor1/RConn2 -- V+/RConn1
  Current Sensor1/RConn1 -- PS-Simulink Converter 3/LConn1 -- PS Product/LConn1 -- I_out/RConn1
  pow_out/RConn1 -- PS Product/RConn1 -- PS-Simulink Converter 4/LConn1

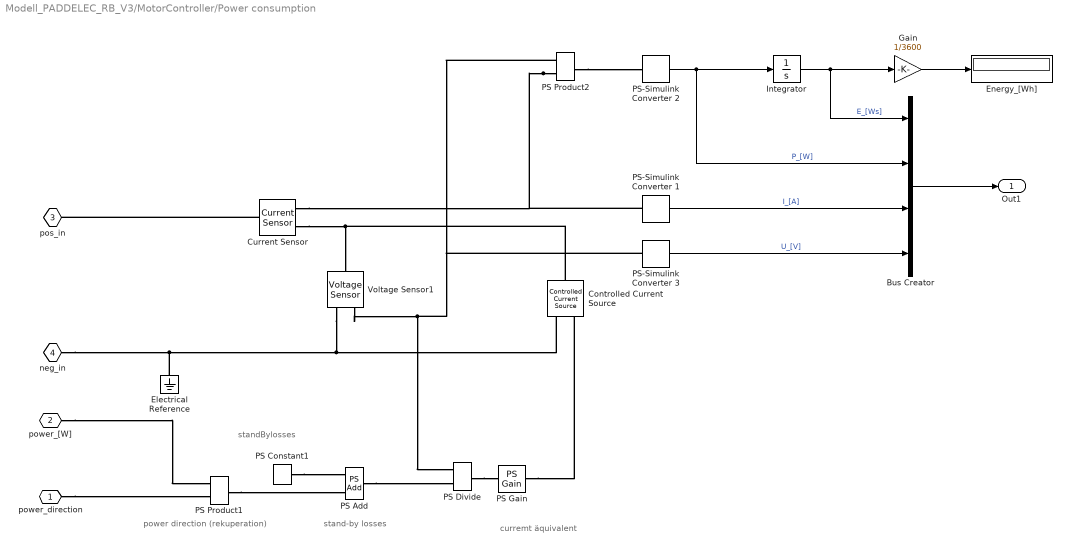
== system Modell_PADDELEC_RB_V3/MotorController/Power consumption ==
  note: standBylosses
  note: curremt äquivalent
  note: stand-by losses
  note: power direction (rekuperation)
  Bus Creator : BusCreator  Inputs=4
  Controlled Current Source : fl_lib/Electrical/Electrical Sources/Controlled Current Source
      settings: LogSimulationData=on
  Current Sensor : fl_lib/Electrical/Electrical Sensors/Current Sensor
  Electrical Reference : fl_lib/Electrical/Electrical Elements/Electrical Reference
  Energy_[Wh] : Display
  Gain : Gain  Gain=1/3600
  Integrator : Integrator
  PS Add : fl_lib/Physical Signals/Functions/PS Add
  PS Constant1 : fl_lib/Physical Signals/Sources/PS Constant  constant=MotorECU.stand_by_losses W
  PS Divide : fl_lib/Physical Signals/Functions/PS Divide
      settings: SourceProductName=Simscape  SourceProductBaseCode=SS
  PS Gain : fl_lib/Physical Signals/Functions/PS Gain  gain=-1
  PS Product1 : fl_lib/Physical Signals/Functions/PS Product
      settings: SourceProductName=Simscape
  PS Product2 : fl_lib/Physical Signals/Functions/PS Product
      settings: SourceProductName=Simscape
  PS-Simulink Converter 1 : nesl_utility/PS-Simulink Converter  PhysicalDomain=network_engine_domain  SubClassName=ps_output  LeftPortType=input  RightPortType=output  PseudoPeriodic=off  Frequencies=[]  Unit=A  AffineConversion=off
  PS-Simulink Converter 2 : nesl_utility/PS-Simulink Converter  PhysicalDomain=network_engine_domain  SubClassName=ps_output  LeftPortType=input  RightPortType=output  PseudoPeriodic=off  Frequencies=[]  Unit=W  AffineConversion=off
  PS-Simulink Converter 3 : nesl_utility/PS-Simulink Converter  PhysicalDomain=network_engine_domain  SubClassName=ps_output  LeftPortType=input  RightPortType=output  PseudoPeriodic=off  Frequencies=[]  Unit=V  AffineConversion=off
  Voltage Sensor1 : fl_lib/Electrical/Electrical Sensors/Voltage Sensor
  power_direction : PMIOPort  Side=Left
  power_[W] : PMIOPort  Port=2  Side=Left
  pos_in : PMIOPort  Port=3  Side=Left
  neg_in : PMIOPort  Port=4  Side=Left
  Out1 : Outport
  wires:
  PS-Simulink Converter 2/1 -> Integrator/1, Bus Creator/2  "P_[W]"
  Integrator/1 -> Gain/1, Bus Creator/1  "E_[Ws]"
  Bus Creator/1 -> Out1/1
  PS-Simulink Converter 3/1 -> Bus Creator/4  "U_[V]"
  PS-Simulink Converter 1/1 -> Bus Creator/3  "I_[A]"
  Gain/1 -> Energy_[Wh]/1
  connections:
  PS Gain/RConn1 -- Controlled Current Source/RConn1
  Electrical Reference/LConn1 -- neg_in/RConn1 -- Controlled Current Source/RConn2 -- Voltage Sensor1/RConn2
  power_direction/RConn1 -- PS Product1/LConn2
  PS Product1/RConn1 -- PS Add/LConn2
  PS Constant1/RConn1 -- PS Add/LConn1
  power_[W]/RConn1 -- PS Product1/LConn1
  PS Divide/RConn1 -- PS Gain/LConn1
  Voltage Sensor1/RConn1 -- PS Product2/LConn1 -- PS-Simulink Converter 3/LConn1 -- PS Divide/LConn2
  PS Product2/LConn2 -- PS-Simulink Converter 1/LConn1 -- Current Sensor/RConn1
  PS Product2/RConn1 -- PS-Simulink Converter 2/LConn1
  Current Sensor/RConn2 -- Controlled Current Source/LConn1 -- Voltage Sensor1/LConn1
  Current Sensor/LConn1 -- pos_in/RConn1
  PS Add/RConn1 -- PS Divide/LConn1

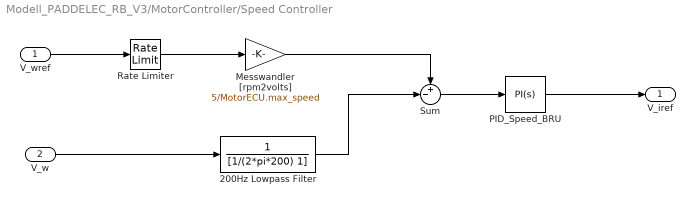
== system Modell_PADDELEC_RB_V3/MotorController/Speed Controller ==
  V_wref : Inport
  V_w : Inport  Port=2
  200Hz Lowpass Filter : TransferFcn  Denominator=[1/(2*pi*200) 1]
  Messwandler [rpm2volts] : Gain  Gain=5/MotorECU.max_speed
  PID_Speed_BRU : simulink/Continuous/PID Controller  Controller=PI  Form=Parallel  TimeDomain=Continuous-time  SampleTime=-1  IntegratorMethod=Forward Euler  FilterMethod=Forward Euler  ControllerParametersSource=internal  P=MotorECU.Speed_Prop  I=MotorECU.Speed_Int  D=0  UseFilter=on  N=100  TunerSelectOption=Transfer Function Based (PID Tuner App)  InitialConditionSource=internal  InitialConditionForIntegrator=0  InitialConditionForFilter=0  DifferentiatorICPrevScaledInput=0  ExternalReset=none  TrackingMode=off  Kt=1  LimitOutput=off  UpperSaturationLimit=10  LowerSaturationLimit=-10  LinearizeAsGain=on  AntiWindupMode=none  Kb=1  POutMin=[]  POutMax=[]  IOutMin=[]  IOutMax=[]  DOutMin=[]  DOutMax=[]  NOutMin=[]  NOutMax=[]  SumOutMin=[]  SumOutMax=[]  SaturationOutMin=[]  SaturationOutMax=[]  PParamMin=[]  PParamMax=[]  IParamMin=[]  IParamMax=[]  DParamMin=[]  DParamMax=[]  NParamMin=[]  NParamMax=[]  KbParamMin=[]  KbParamMax=[]  KtParamMin=[]  KtParamMax=[]  KbOutMin=[]  KbOutMax=[]  KtOutMin=[]  KtOutMax=[]  IntegratorOutMin=[]  IntegratorOutMax=[]  FilterOutMin=[]  FilterOutMax=[]  SumI1OutMin=[]  SumI1OutMax=[]  SumI2OutMin=[]  SumI2OutMax=[]  SumI3OutMin=[]  SumI3OutMax=[]  SumI4OutMin=[]  SumI4OutMax=[]  SumDOutMin=[]  SumDOutMax=[]  DifferentiatorOutMin=[]  DifferentiatorOutMax=[]  FilterDiffOutCoefMin=[]  FilterDiffOutCoefMax=[]  ReciprocalOutMin=[]  ReciprocalOutMax=[]  SumDenOutMin=[]  SumDenOutMax=[]  SumNumOutMin=[]  SumNumOutMax=[]  DivideOutMin=[]  DivideOutMax=[]  IntegratorContinuousStateAttributes=''  IntegratorStateMustResolveToSignalObject=off  IntegratorRTWStateStorageClass=Auto  FilterContinuousStateAttributes=''  FilterStateMustResolveToSignalObject=off  FilterRTWStateStorageClass=Auto  ParallelPVariant=InternalParameters  IdealPVariant=Disabled  IVariant=InternalParameters  DVariant=Disabled  IntegratorVariant=Continuous  SatVariant=Disabled  AWVariant=Passthrough  PCopyVariant=Disabled  TRVariant=Disabled  FdbkBlocksVariant=Forward  IdealPFdbkVariant=Disabled  SatFdbkVariant=Disabled  DerivativeFilterVariant=Disabled  NVariant=Disabled  NCopyVariant=Disabled_SignalSpec  FilterICVariant=Disabled  IntegratorICVariant=InternalICs  ExternalResetVariant=Disabled  TRSumVariant=Passthrough  SumFdbkVariant=Disabled  SumVariant=Sum_PI
  Rate Limiter : RateLimiter  RisingSlewLimit=MotorECU.max_speed/MotorECU.slew_rate_up  FallingSlewLimit=-MotorECU.max_speed/MotorECU.slew_rate_down  SampleTimeMode=inherited
  Sum : Sum  Inputs=+-|
  V_iref : Outport
  wires:
  PID_Speed_BRU/1 -> V_iref/1
  Sum/1 -> PID_Speed_BRU/1
  V_w/1 -> 200Hz Lowpass Filter/1
  V_wref/1 -> Rate Limiter/1
  Rate Limiter/1 -> Messwandler [rpm2volts]/1
  Messwandler [rpm2volts]/1 -> Sum/1
  200Hz Lowpass Filter/1 -> Sum/2

== system Modell_PADDELEC_RB_V3/iPADDLE/MEMS_Data ==
  Beta_Pad : Constant  Value=0
  Bus Creator : BusCreator  Inputs=1
  MEMS : Outport
  wires:
  Beta_Pad/1 -> Bus Creator/1
  Bus Creator/1 -> MEMS/1

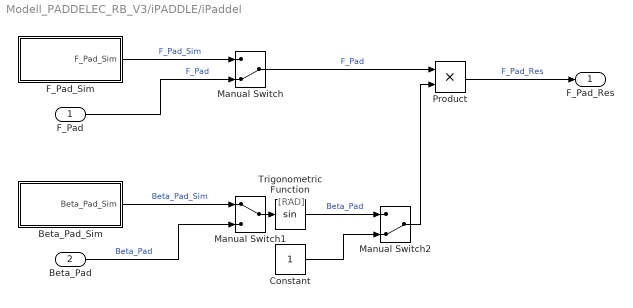
== system Modell_PADDELEC_RB_V3/iPADDLE/iPaddel ==
  note: [RAD]
  F_Pad : Inport
  Beta_Pad : Inport  Port=2
  Beta_Pad_Sim : Subsystem
  Constant : Constant
  F_Pad_Sim : Subsystem
  Manual Switch : ManualSwitch  CurrentSetting=0
  Manual Switch1 : ManualSwitch
  Manual Switch2 : ManualSwitch  CurrentSetting=0
  Product : Product
  Trigonometric Function : Trigonometry
  F_Pad_Res : Outport  VectorParamsAs1DForOutWhenUnconnected=off
  wires:
  F_Pad/1 -> Manual Switch/2  "F_Pad"
  Beta_Pad/1 -> Manual Switch1/2  "Beta_Pad"
  Product/1 -> F_Pad_Res/1  "F_Pad_Res"
  Trigonometric Function/1 -> Manual Switch2/1  "Beta_Pad"
  F_Pad_Sim/1(F_Pad_Sim) -> Manual Switch/1  "F_Pad_Sim"
  Manual Switch/1 -> Product/1  "F_Pad"
  Beta_Pad_Sim/1(Beta_Pad_Sim) -> Manual Switch1/1  "Beta_Pad_Sim"
  Manual Switch1/1 -> Trigonometric Function/1
  Manual Switch2/1 -> Product/2
  Constant/1 -> Manual Switch2/2

== system Modell_PADDELEC_RB_V3/MotorController/Current Controller/SL2V_1 ==
  SL : Inport
  Controlled Voltage Source : fl_lib/Electrical/Electrical Sources/Controlled Voltage Source
  Electrical Reference : fl_lib/Electrical/Electrical Elements/Electrical Reference
  Simulink-PS Converter : nesl_utility/Simulink-PS Converter  PhysicalDomain=network_engine_domain  SubClassName=ps_input  LeftPortType=input  RightPortType=output  PseudoPeriodic=off  Frequencies=[]  NoiseDistribution=none  NoiseParameters=[]  Unit=V  AffineConversion=off  FilteringAndDerivatives=zero  SimscapeFilterOrder=1  InputFilterTimeConstant=.001  UdotUserProvided=0
  V : PMIOPort  Side=Right
  wires:
  SL/1 -> Simulink-PS Converter/1
  connections:
  Simulink-PS Converter/RConn1 -- Controlled Voltage Source/RConn1
  V/RConn1 -- Controlled Voltage Source/LConn1
  Electrical Reference/LConn1 -- Controlled Voltage Source/RConn2

== system Modell_PADDELEC_RB_V3/MotorController/Current Controller/SL2V_2 ==
  SL : Inport
  Controlled Voltage Source : fl_lib/Electrical/Electrical Sources/Controlled Voltage Source
  Electrical Reference : fl_lib/Electrical/Electrical Elements/Electrical Reference
  Simulink-PS Converter : nesl_utility/Simulink-PS Converter  PhysicalDomain=network_engine_domain  SubClassName=ps_input  LeftPortType=input  RightPortType=output  PseudoPeriodic=off  Frequencies=[]  NoiseDistribution=none  NoiseParameters=[]  Unit=V  AffineConversion=off  FilteringAndDerivatives=zero  SimscapeFilterOrder=1  InputFilterTimeConstant=.001  UdotUserProvided=0
  V : PMIOPort  Side=Right
  wires:
  SL/1 -> Simulink-PS Converter/1
  connections:
  Electrical Reference/LConn1 -- Controlled Voltage Source/RConn2
  V/RConn1 -- Controlled Voltage Source/LConn1
  Simulink-PS Converter/RConn1 -- Controlled Voltage Source/RConn1

== system Modell_PADDELEC_RB_V3/MotorController/PWM & H-Bridge/PWM Scope ==
  Electrical Reference1 : fl_lib/Electrical/Electrical Elements/Electrical Reference
  PS-Simulink Converter 2 : nesl_utility/PS-Simulink Converter  PhysicalDomain=network_engine_domain  SubClassName=ps_output  LeftPortType=input  RightPortType=output  PseudoPeriodic=off  Frequencies=[]  Unit=V  AffineConversion=off
  REV : Scope
  Voltage Sensor : fl_lib/Electrical/Electrical Sensors/Voltage Sensor
  u : PMIOPort  Side=Left
  wires:
  PS-Simulink Converter 2/1 -> REV/1
  connections:
  Voltage Sensor/RConn2 -- Electrical Reference1/LConn1
  Voltage Sensor/RConn1 -- PS-Simulink Converter 2/LConn1
  u/RConn1 -- Voltage Sensor/LConn1

== system Modell_PADDELEC_RB_V3/MotorController/PWM & H-Bridge/REV Scope ==
  Electrical Reference1 : fl_lib/Electrical/Electrical Elements/Electrical Reference
  PS-Simulink Converter 2 : nesl_utility/PS-Simulink Converter  PhysicalDomain=network_engine_domain  SubClassName=ps_output  LeftPortType=input  RightPortType=output  PseudoPeriodic=off  Frequencies=[]  Unit=V  AffineConversion=off
  REV : Scope
  Voltage Sensor : fl_lib/Electrical/Electrical Sensors/Voltage Sensor
  u : PMIOPort  Side=Left
  wires:
  PS-Simulink Converter 2/1 -> REV/1
  connections:
  u/RConn1 -- Voltage Sensor/LConn1
  Voltage Sensor/RConn1 -- PS-Simulink Converter 2/LConn1
  Voltage Sensor/RConn2 -- Electrical Reference1/LConn1

== system Modell_PADDELEC_RB_V3/iPADDLE/iPaddel/Beta_Pad_Sim ==
  Add : Sum
  "Beta_Pad_Sim " : Sin  Amplitude=45  Frequency=3  SampleTime=0
  Constant : Constant  Value=0
  Constant1 : Constant  Value=45
  Gain : Gain  Gain=pi/180
  Switch : Switch
  Beta_Pad_Sim : Outport
  wires:
  Constant/1 -> Switch/3
  Gain/1 -> Beta_Pad_Sim/1
  "Beta_Pad_Sim "/1 -> Switch/2, Switch/1
  Switch/1 -> Add/1
  Add/1 -> Gain/1
  Constant1/1 -> Add/2

== system Modell_PADDELEC_RB_V3/iPADDLE/iPaddel/F_Pad_Sim ==
  Constant : Constant  Value=0
  "F_Pad_Sim " : Sin  Amplitude=80  Frequency=3  SampleTime=0
  Switch : Switch
  F_Pad_Sim : Outport
  wires:
  "F_Pad_Sim "/1 -> Switch/2, Switch/1
  Switch/1 -> F_Pad_Sim/1
  Constant/1 -> Switch/3
